simulink model "model"  (R2021b)
settings: Solver=VariableStepAuto  StartTime=0.0  StopTime=10.0  RelTol=1e-3
undefined symbols (not defined in the file): Newton, Raphson
libraries: simulink x3, slpidlib x2
settings Model: Creator=O  LastModifiedBy=wangzixuan

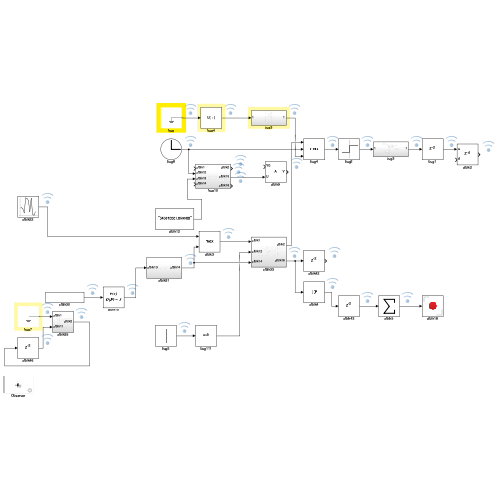
[thumbnail: Simulink's stored preview of the top-level diagram]
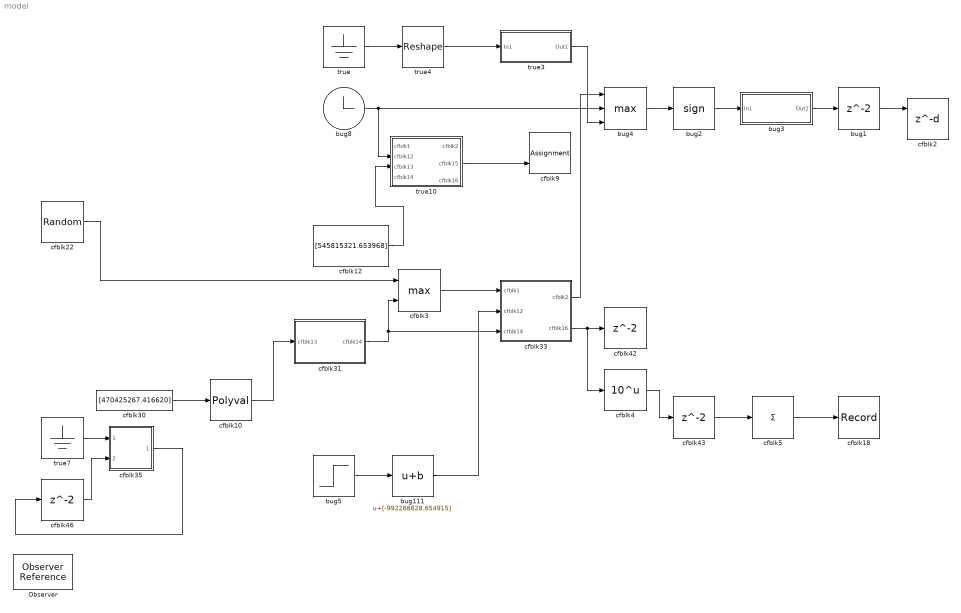
== system model ==
  Observer : ObserverReference  ObserverModelName=sampleModel714_pp_5_1_difftest_Observer1
  bug1 : Delay  SampleTime=1
  bug111 : Bias  Bias=[-992268628.654915]
  bug2 : Signum
  bug3 : Subsystem
  bug4 : MinMax  Function=max  Inputs=3  OutDataTypeStr=double
  bug5 : Step  Time=[40.000000]  Before=[-68333763.593446]  After=[671371691.307936]  SampleTime=0
  bug8 : Clock
  cfblk10 : Polyval  Coefs=[ +2.081618890e-019, -1.441693666e-014, +4.719686976e-010, -8.536869453e-006, +1.621573104e-001, -8.087801117e+001 ]
  cfblk12 : Constant  Value=[545815321.653968]  OutDataTypeStr=double  SampleTime=1
  cfblk18 : Record  FileSettingsInternal="{\"entries\":[{\"content\":{\"excelSettings\":{\"content\":{},\"type\":\"Streamout.ExcelSettings\"}},\"type\":\"Streamout.FileSettingStorage\",\"uuid\":\"378b8976-508a-4c36-8cfc-804270fadb91\"}],\"packageUris\":[\"http://schema.mathworks.com/mf0/streamout_blocks/R2020a\"],\"version\":\"1.0\"}"  SignalsInternal="{\"entries\":[{\"content\":{\"signals\":[{\"content\":{\"blockPath\":[\"sampleModel714_pp_5_1_difftest/cfblk18\"],\"channel\":[],\"dimensions\":[1],\"domain\":\"sampleModel714_pp_5_1_difftest/cfblk18\",\"lineColor\":\"#ff13a6\",\"plots\":[1],\"port\":1,\"sid\":[\"\"],\"signalID\":424995,\"signalName\":\"cfblk5\"},\"type\":\"RecordBlkView.Signal\",\"uuid\":\"6ae9b17c-bea1-45aa-a5b0-6a23d3646b80\"}]},\"type\":\"RecordBlkView.InputSignals\",\"uuid\":\"94cf21f0-f853-4485-8966-5fcfe03de0c2\"}],\"packageUris\":[\"http://schema.mathworks.com/mf0/streamout_blocks/R2020a\"],\"version\":\"1.0\"}"  VisualizationBindings="{\"sparklinesplugin\":{\"info\":[{\"bindingParametersList\":[],\"subplotID\":1}]}}"
  cfblk2 : Delay  DelayLengthSource=Input port  SampleTime=1
      settings: InputPortMap=u0,p1
  cfblk22 : RandomNumber  Mean=[-90222.913364]  Variance=[78530.805883]  Seed=[550576936.000000]  SampleTime=0.1
  cfblk3 : MinMax  Function=max  Inputs=2  OutDataTypeStr=double
  cfblk30 : Constant  Value=[470425267.416620]  OutDataTypeStr=double  SampleTime=1
  cfblk31 : Subsystem
  cfblk33 : Subsystem
  cfblk35 : Subsystem
  cfblk4 : Math  Operator=10^u  OutDataTypeStr=double  SaturateOnIntegerOverflow=on
  cfblk42 : Delay  SampleTime=1
  cfblk43 : Delay  SampleTime=1
  cfblk46 : Delay  SampleTime=1
  cfblk5 : Sum  Inputs=+  OutDataTypeStr=double
  cfblk9 : Assignment  DiagnosticForDimensions=Warning  IndexOptions=Index vector (dialog)  Indices=1  OutputSizes=1
  true : Ground
  true10 : Subsystem
  true3 : Subsystem
  true4 : Reshape
  true7 : Ground
  wires:
  cfblk4/1 -> cfblk43/1
  cfblk31/1(cfblk14) -> cfblk3/2, cfblk33/3(cfblk14)
  cfblk33/2(cfblk16) -> cfblk42/1, cfblk4/1
  bug4/1 -> bug2/1
  cfblk33/1(cfblk2) -> bug4/1
  true3/1(Out1) -> bug4/3
  cfblk22/1 -> cfblk3/1
  bug1/1 -> cfblk2/1
  cfblk30/1 -> cfblk10/1
  cfblk10/1 -> cfblk31/1(cfblk13)
  bug8/1 -> bug4/2, true10/2(cfblk12)
  cfblk5/1 -> cfblk18/1
  true4/1 -> true3/1(In1)
  true7/1 -> cfblk35/1(cfblk1)
  bug5/1 -> bug111/1
  cfblk35/1(cfblk2) -> cfblk46/1
  cfblk43/1 -> cfblk5/1
  true/1 -> true4/1
  cfblk46/1 -> cfblk35/2(cfblk11)
  bug111/1 -> cfblk33/2(cfblk12)
  bug2/1 -> bug3/1(In1)
  true10/2(cfblk15) -> cfblk9/2
  cfblk3/1 -> cfblk33/1(cfblk1)
  bug3/1(Out1) -> bug1/1
  cfblk12/1 -> true10/3(cfblk13)

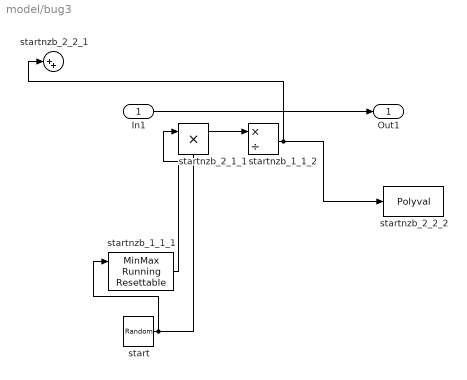
== system model/bug3 ==
  In1 : Inport
  start : RandomNumber  SampleTime=0.1
  startnzb_1_1_1 : simulink/Math Operations/MinMax Running Resettable  Function=min  vinit=0.0
  startnzb_1_1_2 : Product  Inputs=*/
  startnzb_2_1_1 : Product
  startnzb_2_2_1 : Sum  Inputs=|++
  startnzb_2_2_2 : Polyval  Coefs=[ +2.081618890e-019, -1.441693666e-014, +4.719686976e-010, -8.536869453e-006, +1.621573104e-001, -8.087801117e+001 ]
  Out1 : Outport
  wires:
  In1/1 -> Out1/1
  start/1 -> startnzb_1_1_1/1, startnzb_1_1_2/1
  startnzb_1_1_1/1 -> startnzb_2_1_1/1
  startnzb_1_1_2/1 -> startnzb_2_2_1/1, startnzb_2_2_2/1

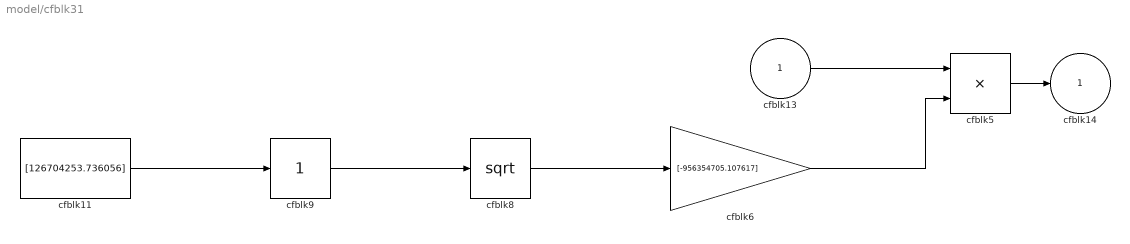
== system model/cfblk31 ==
  cfblk13 : Inport
  cfblk11 : Constant  Value=[126704253.736056]  OutDataTypeStr=double  SampleTime=1
  cfblk5 : Product  Inputs=**  OutDataTypeStr=double
  cfblk6 : Gain  Gain=[-956354705.107617]  OutDataTypeStr=double
  cfblk8 : Sqrt  OutDataTypeStr=double  SaturateOnIntegerOverflow=on
  cfblk9 : simulink/Math Operations/Slider Gain  gain=1  low=0  high=2
  cfblk14 : Outport
  wires:
  cfblk5/1 -> cfblk14/1
  cfblk6/1 -> cfblk5/2
  cfblk13/1 -> cfblk5/1
  cfblk8/1 -> cfblk6/1
  cfblk9/1 -> cfblk8/1
  cfblk11/1 -> cfblk9/1

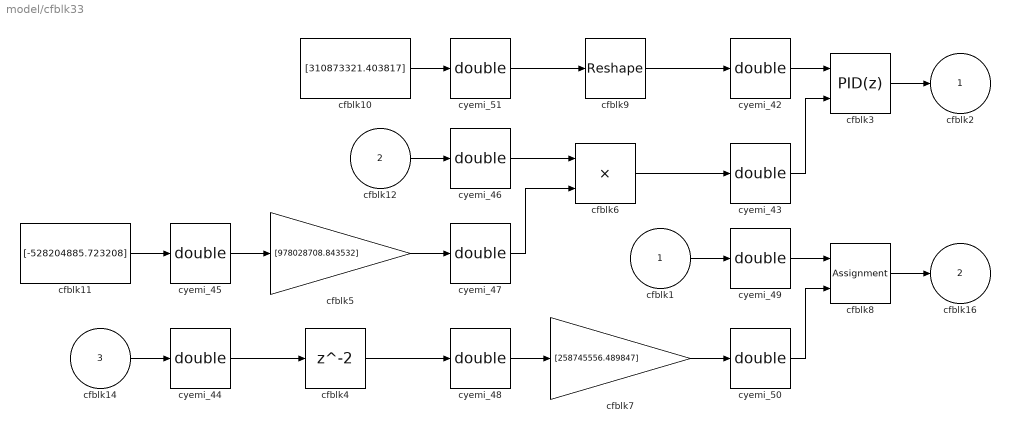
== system model/cfblk33 ==
  cfblk1 : Inport
  cfblk12 : Inport  Port=2
  cfblk14 : Inport  Port=3
  cfblk10 : Constant  Value=[310873321.403817]  OutDataTypeStr=double  SampleTime=1
  cfblk11 : Constant  Value=[-528204885.723208]  OutDataTypeStr=double  SampleTime=1
  cfblk3 : slpidlib/PID Controller (2DOF)  Controller=PID  Form=Parallel  TimeDomain=Discrete-time  UseExternalTs=off  SampleTime=1  IntegratorMethod=Forward Euler  FilterMethod=Forward Euler  ControllerParametersSource=internal  P=1  I=1  D=0  UseFilter=on  N=100  b=1  c=1  TunerSelectOption=Transfer Function Based (PID Tuner App)  InitialConditionSource=internal  InitialConditionForIntegrator=0  InitialConditionForFilter=0  DifferentiatorICPrevScaledInput=0  ExternalReset=none  TrackingMode=off  Kt=1  LimitOutput=off  SatLimitsSource=internal  UpperSaturationLimit=inf  LowerSaturationLimit=-inf  LinearizeAsGain=off  AntiWindupMode=none  Kb=1  POutMin=[]  POutMax=[]  IOutMin=[]  IOutMax=[]  DOutMin=[]  DOutMax=[]  NOutMin=[]  NOutMax=[]  bOutMin=[]  bOutMax=[]  cOutMin=[]  cOutMax=[]  SumOutMin=[]  SumOutMax=[]  SaturationOutMin=[]  SaturationOutMax=[]  PParamMin=[]  PParamMax=[]  IParamMin=[]  IParamMax=[]  DParamMin=[]  DParamMax=[]  NParamMin=[]  NParamMax=[]  bParamMin=[]  bParamMax=[]  cParamMin=[]  cParamMax=[]  KbParamMin=[]  KbParamMax=[]  KtParamMin=[]  KtParamMax=[]  KbOutMin=[]  KbOutMax=[]  KtOutMin=[]  KtOutMax=[]  IntegratorOutMin=[]  IntegratorOutMax=[]  FilterOutMin=[]  FilterOutMax=[]  SumI1OutMin=[]  SumI1OutMax=[]  SumI2OutMin=[]  SumI2OutMax=[]  SumI3OutMin=[]  SumI3OutMax=[]  SumI4OutMin=[]  SumI4OutMax=[]  SumDOutMin=[]  SumDOutMax=[]  Sum1OutMin=[]  Sum1OutMax=[]  Sum2OutMin=[]  Sum2OutMax=[]  Sum3OutMin=[]  Sum3OutMax=[]  DifferentiatorOutMin=[]  DifferentiatorOutMax=[]  FilterDiffOutCoefMin=[]  FilterDiffOutCoefMax=[]  ReciprocalOutMin=[]  ReciprocalOutMax=[]  SumDenOutMin=[]  SumDenOutMax=[]  SumNumOutMin=[]  SumNumOutMax=[]  DivideOutMin=[]  DivideOutMax=[]  UdiffTsProdOutMin=[]  UdiffTsProdOutMax=[]  NTsProdOutMin=[]  NTsProdOutMax=[]  UintegralTsProdOutMin=[]  UintegralTsProdOutMax=[]  UngainTsProdOutMin=[]  UngainTsProdOutMax=[]  IntegratorContinuousStateAttributes=''  IntegratorStateMustResolveToSignalObject=off  IntegratorRTWStateStorageClass=Auto  FilterContinuousStateAttributes=''  FilterStateMustResolveToSignalObject=off  FilterRTWStateStorageClass=Auto  ParallelPVariant=InternalParameters  IdealPVariant=Disabled  IVariant=InternalParameters  DVariant=InternalParameters  bVariant=InternalParameters  cVariant=InternalParameters  IntegratorVariant=Discrete  SatVariant=Disabled  AWVariant=Passthrough  PCopyVariant=Disabled  TRVariant=Disabled  FdbkBlocksVariant=Forward  IdealPFdbkVariant=Disabled  SatFdbkVariant=Disabled  DerivativeFilterVariant=ForwardEulerFilter  NVariant=InternalParameters  NCopyVariant=Disabled  FilterICVariant=InternalICsFilter  IntegratorICVariant=InternalICs  ExternalResetVariant=Disabled  TRSumVariant=Passthrough  SumFdbkVariant=Disabled  SumVariant=Sum_PID  TsampFilterVariant=InternalTs  TsampNgainVariant=Passthrough  TsampIntegralVariant=Passthrough  ExternalSaturationOutDataTypeStr=Inherit: Same as second input
      settings: SourceProductBaseCode=SL
  cfblk4 : Delay  SampleTime=1
  cfblk5 : Gain  Gain=[978028708.843532]  OutDataTypeStr=double
  cfblk6 : Product  Inputs=**  OutDataTypeStr=double
  cfblk7 : Gain  Gain=[258745556.489847]  OutDataTypeStr=double
  cfblk8 : Assignment  DiagnosticForDimensions=Warning  IndexOptions=Index vector (dialog)  Indices=1  OutputSizes=1
  cfblk9 : Reshape
  cyemi_{42..51} (10 alike) : DataTypeConversion  OutDataTypeStr=double
  cfblk2 : Outport
  cfblk16 : Outport  Port=2
  wires:
  cfblk3/1 -> cfblk2/1
  cfblk8/1 -> cfblk16/1
  cfblk6/1 -> cyemi_43/1
  cyemi_44/1 -> cfblk4/1
  cfblk9/1 -> cyemi_42/1
  cfblk14/1 -> cyemi_44/1
  cyemi_45/1 -> cfblk5/1
  cfblk11/1 -> cyemi_45/1
  cyemi_46/1 -> cfblk6/1
  cyemi_48/1 -> cfblk7/1
  cfblk5/1 -> cyemi_47/1
  cfblk7/1 -> cyemi_50/1
  cfblk4/1 -> cyemi_48/1
  cfblk10/1 -> cyemi_51/1
  cyemi_49/1 -> cfblk8/1
  cyemi_43/1 -> cfblk3/2
  cfblk1/1 -> cyemi_49/1
  cyemi_42/1 -> cfblk3/1
  cyemi_50/1 -> cfblk8/2
  cyemi_47/1 -> cfblk6/2
  cyemi_51/1 -> cfblk9/1
  cfblk12/1 -> cyemi_46/1

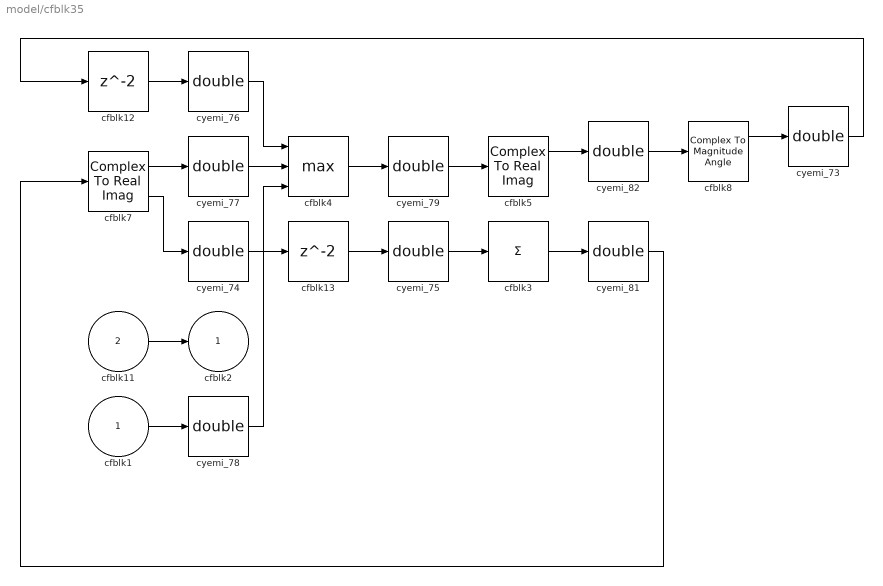
== system model/cfblk35 ==
  cfblk1 : Inport
  cfblk11 : Inport  Port=2
  cfblk12 : Delay  SampleTime=1
  cfblk13 : Delay  SampleTime=1
  cfblk3 : Sum  Inputs=+  OutDataTypeStr=double
  cfblk4 : MinMax  Function=max  Inputs=3  OutDataTypeStr=double
  cfblk5 : ComplexToRealImag
  cfblk7 : ComplexToRealImag
  cfblk8 : ComplexToMagnitudeAngle
  cyemi_{73..79,81..82} (9 alike) : DataTypeConversion  OutDataTypeStr=double
  cfblk2 : Outport
  wires:
  cfblk11/1 -> cfblk2/1
  cyemi_73/1 -> cfblk12/1
  cfblk8/1 -> cyemi_73/1
  cyemi_74/1 -> cfblk13/1
  cfblk7/2 -> cyemi_74/1
  cyemi_75/1 -> cfblk3/1
  cfblk13/1 -> cyemi_75/1
  cyemi_76/1 -> cfblk4/1
  cfblk12/1 -> cyemi_76/1
  cyemi_77/1 -> cfblk4/2
  cfblk7/1 -> cyemi_77/1
  cyemi_78/1 -> cfblk4/3
  cfblk1/1 -> cyemi_78/1
  cfblk4/1 -> cyemi_79/1
  cyemi_81/1 -> cfblk7/1
  cfblk3/1 -> cyemi_81/1
  cyemi_82/1 -> cfblk8/1
  cfblk5/1 -> cyemi_82/1
  cyemi_79/1 -> cfblk5/1

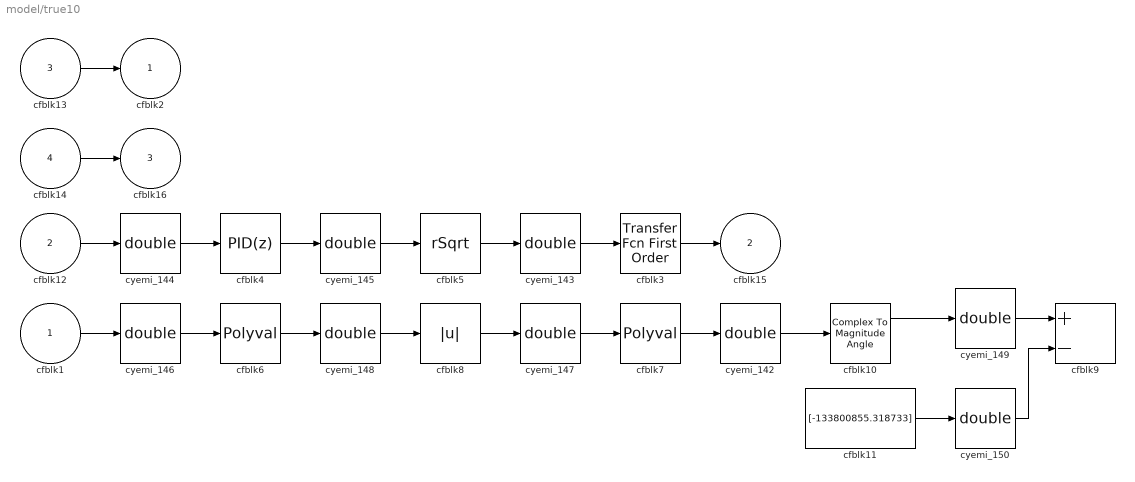
== system model/true10 ==
  cfblk1 : Inport
  cfblk12 : Inport  Port=2
  cfblk13 : Inport  Port=3
  cfblk14 : Inport  Port=4
  cfblk10 : ComplexToMagnitudeAngle
  cfblk11 : Constant  Value=[-133800855.318733]  OutDataTypeStr=double  SampleTime=1
  cfblk3 : simulink/Discrete/Transfer Fcn First Order  PoleZ=0.95  ICPrevOutput=0.0  DoSatur=off
  cfblk4 : slpidlib/PID Controller  Controller=PID  Form=Parallel  TimeDomain=Discrete-time  UseExternalTs=off  SampleTime=1  IntegratorMethod=Forward Euler  FilterMethod=Forward Euler  ControllerParametersSource=internal  P=1  I=1  D=0  UseFilter=on  N=100  TunerSelectOption=Transfer Function Based (PID Tuner App)  InitialConditionSource=internal  InitialConditionForIntegrator=0  InitialConditionForFilter=0  DifferentiatorICPrevScaledInput=0  ExternalReset=none  TrackingMode=off  Kt=1  LimitOutput=off  SatLimitsSource=internal  UpperSaturationLimit=inf  LowerSaturationLimit=-inf  LinearizeAsGain=off  AntiWindupMode=none  Kb=1  POutMin=[]  POutMax=[]  IOutMin=[]  IOutMax=[]  DOutMin=[]  DOutMax=[]  NOutMin=[]  NOutMax=[]  SumOutMin=[]  SumOutMax=[]  SaturationOutMin=[]  SaturationOutMax=[]  PParamMin=[]  PParamMax=[]  IParamMin=[]  IParamMax=[]  DParamMin=[]  DParamMax=[]  NParamMin=[]  NParamMax=[]  KbParamMin=[]  KbParamMax=[]  KtParamMin=[]  KtParamMax=[]  KbOutMin=[]  KbOutMax=[]  KtOutMin=[]  KtOutMax=[]  IntegratorOutMin=[]  IntegratorOutMax=[]  FilterOutMin=[]  FilterOutMax=[]  SumI1OutMin=[]  SumI1OutMax=[]  SumI2OutMin=[]  SumI2OutMax=[]  SumI3OutMin=[]  SumI3OutMax=[]  SumI4OutMin=[]  SumI4OutMax=[]  SumDOutMin=[]  SumDOutMax=[]  DifferentiatorOutMin=[]  DifferentiatorOutMax=[]  FilterDiffOutCoefMin=[]  FilterDiffOutCoefMax=[]  ReciprocalOutMin=[]  ReciprocalOutMax=[]  SumDenOutMin=[]  SumDenOutMax=[]  SumNumOutMin=[]  SumNumOutMax=[]  DivideOutMin=[]  DivideOutMax=[]  UdiffTsProdOutMin=[]  UdiffTsProdOutMax=[]  NTsProdOutMin=[]  NTsProdOutMax=[]  UintegralTsProdOutMin=[]  UintegralTsProdOutMax=[]  UngainTsProdOutMin=[]  UngainTsProdOutMax=[]  IntegratorContinuousStateAttributes=''  IntegratorStateMustResolveToSignalObject=off  IntegratorRTWStateStorageClass=Auto  FilterContinuousStateAttributes=''  FilterStateMustResolveToSignalObject=off  FilterRTWStateStorageClass=Auto  ParallelPVariant=InternalParameters  IdealPVariant=Disabled  IVariant=InternalParameters  DVariant=InternalParameters  IntegratorVariant=Discrete  SatVariant=Disabled  AWVariant=Passthrough  PCopyVariant=Disabled  TRVariant=Disabled  FdbkBlocksVariant=Forward  IdealPFdbkVariant=Disabled  SatFdbkVariant=Disabled  DerivativeFilterVariant=ForwardEulerFilter  NVariant=InternalParameters  NCopyVariant=Disabled  FilterICVariant=InternalICsFilter  IntegratorICVariant=InternalICs  ExternalResetVariant=Disabled  TRSumVariant=Passthrough  SumFdbkVariant=Disabled  SumVariant=Sum_PID  TsampFilterVariant=InternalTs  TsampNgainVariant=Passthrough  TsampIntegralVariant=Passthrough  ExternalSaturationOutDataTypeStr=Inherit: Same as second input
  cfblk5 : Sqrt  Operator=rSqrt  OutDataTypeStr=double  AlgorithmType=Newton-Raphson  SaturateOnIntegerOverflow=on
  cfblk6 : Polyval  Coefs=[ +2.081618890e-019, -1.441693666e-014, +4.719686976e-010, -8.536869453e-006, +1.621573104e-001, -8.087801117e+001 ]
  cfblk7 : Polyval  Coefs=[ +2.081618890e-019, -1.441693666e-014, +4.719686976e-010, -8.536869453e-006, +1.621573104e-001, -8.087801117e+001 ]
  cfblk8 : Abs  OutDataTypeStr=double
  cfblk9 : Sum  Inputs=+-  OutDataTypeStr=double
  cyemi_{142..150} (9 alike) : DataTypeConversion  OutDataTypeStr=double
  cfblk2 : Outport
  cfblk15 : Outport  Port=2
  cfblk16 : Outport  Port=3
  wires:
  cfblk3/1 -> cfblk15/1
  cfblk14/1 -> cfblk16/1
  cyemi_142/1 -> cfblk10/1
  cfblk7/1 -> cyemi_142/1
  cyemi_144/1 -> cfblk4/1
  cfblk4/1 -> cyemi_145/1
  cfblk13/1 -> cfblk2/1
  cfblk1/1 -> cyemi_146/1
  cfblk8/1 -> cyemi_147/1
  cfblk5/1 -> cyemi_143/1
  cyemi_148/1 -> cfblk8/1
  cyemi_149/1 -> cfblk9/1
  cfblk10/1 -> cyemi_149/1
  cfblk6/1 -> cyemi_148/1
  cyemi_145/1 -> cfblk5/1
  cyemi_147/1 -> cfblk7/1
  cyemi_150/1 -> cfblk9/2
  cyemi_143/1 -> cfblk3/1
  cfblk12/1 -> cyemi_144/1
  cyemi_146/1 -> cfblk6/1
  cfblk11/1 -> cyemi_150/1

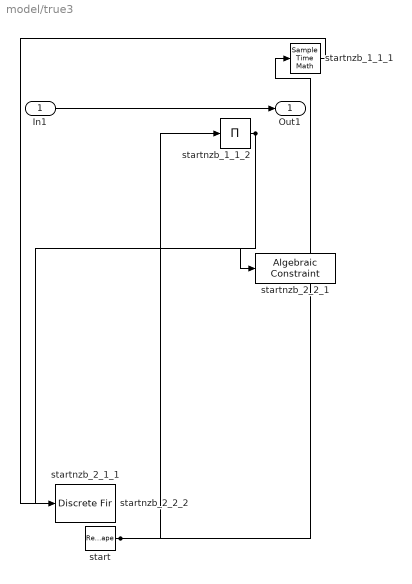
== system model/true3 ==
  In1 : Inport
  start : Reshape
  startnzb_1_1_1 : SampleTimeMath
  startnzb_1_1_2 : Product  Inputs=*
  startnzb_2_1_1 : DiscreteFir
  startnzb_2_2_1 : AlgebraicConstraint
  startnzb_2_2_2 : DiscreteFir
  Out1 : Outport
  wires:
  In1/1 -> Out1/1
  start/1 -> startnzb_1_1_1/1, startnzb_1_1_2/1
  startnzb_1_1_1/1 -> startnzb_2_1_1/1
  startnzb_1_1_2/1 -> startnzb_2_2_1/1, startnzb_2_2_2/1
